simulink model "inv_single_phase"  (R2024b)
settings: Solver=ode1be  StartTime=0.0  StopTime=simlength  FixedStep=ts_sim  MaxStep=ts_sim
undefined symbols (not defined in the file): Adrso, Aresd, Bresd, Cresd, Crso, dead_time, DThs_init, fPWM_INV, freq, frequency_grid, I_FS, ki_i_inv, ki_pll, ki_v_inv, kp_i_inv, kp_pll, kp_v_inv, Ldrso, magnitude, q1kalman, q2kalman, Rkalman, Tambient, ts_inv, ts_zvs, V_FS, w, weigth
libraries: fl_lib x60, nesl_utility x38, ee_lib x9, cstblocks x6
(part 1 of 3)
settings Model: SimulationMode=accelerator  Creator=LTNBDA  LastModifiedBy=dbagn
settings SolverCC: ZeroCrossControl=EnableAll  ZeroCrossAlgorithm=Adaptive  AlgebraicLoopSolver=TrustRegion  SolverResetMethod=Robust  AutoInsertRateTranBlk=on
settings DataIOCC: LimitDataPoints=on  MaxDataPoints=1  SaveFormat=Array  SignalLoggingSaveFormat=ModelDataLogs  SaveOutput=off  SignalLogging=off  DSMLogging=off  SaveTime=off  ReturnWorkspaceOutputs=off
settings OptimizationCC: ExpressionDepthLimit=2147483647  InitFltsAndDblsToZero=on  EfficientMapNaN2IntZero=off  LifeSpan=inf
settings DebuggingCC: SaveWithParameterizedLinksMsg=none  UnderspecifiedInitializationDetection=Classic  MergeDetectMultiDrivingBlocksExec=none  SignalResolutionControl=TryResolveAllWithWarning  SolverPrmCheckMsg=warning  MultiTaskDSMMsg=warning  MultiTaskCondExecSysMsg=none  MultiTaskRateTransMsg=warning  FcnCallInpInsideContextMsg=warning  StateNameClashWarn=warning  SFUnexpectedBacktrackingDiag=warning  SFNoUnconditionalDefaultTransitionDiag=warning  ArithmeticOperatorsInVariantConditions=warning
settings HardwareCC: ProdBitPerLong=64  ProdLargestAtomicFloat=None  ProdIntDivRoundTo=Undefined  ProdEndianess=Unspecified  ProdHWDeviceType=Generic->64-bit Embedded Processor (LP64)  TargetBitPerPointer=64  TargetBitPerSizeT=64  TargetBitPerPtrDiffT=64  TargetLongLongMode=on  TargetIntDivRoundTo=Zero  TargetEndianess=LittleEndian  TargetWordSize=64  TargetHWDeviceType=MATLAB Host  ProdEqTarget=off
settings ModelReferenceCC: EnableRefExpFcnMdlSchedulingChecks=on  PropagateSignalLabelsOutOfModel=off
settings SFSimCC: SimUseLocalCustomCode=off  CustomCodeUndefinedFunction=UseInterfaceOnly
settings RTWCC: RTWUseLocalCustomCode=off  GPUComputeCapability=3.5
settings CodeAppCC: MaxIdLength=128  StateflowObjectComments=on
settings GRTTargetCC: TargetLangStandard=C89/C90 (ANSI)  CombineOutputUpdateFcns=off  GRTInterface=on
settings ConfigComp: CovMetricSettings=dw  CovSaveCumulativeToWorkspaceVar=on  CovSaveSingleToWorkspaceVar=on  CovExternalEMLEnable=off
settings SimscapeCC: SimscapeNormalizeSystem=off

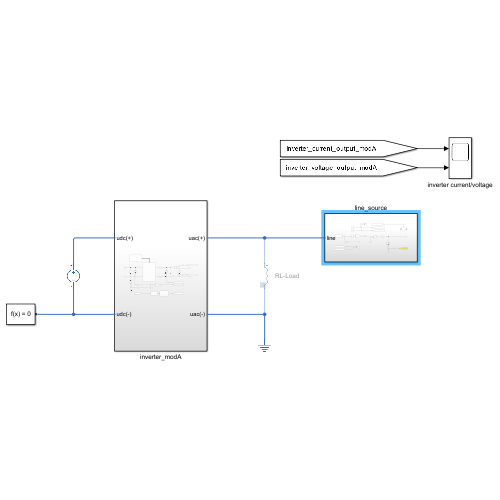
[thumbnail: Simulink's stored preview of the top-level diagram]
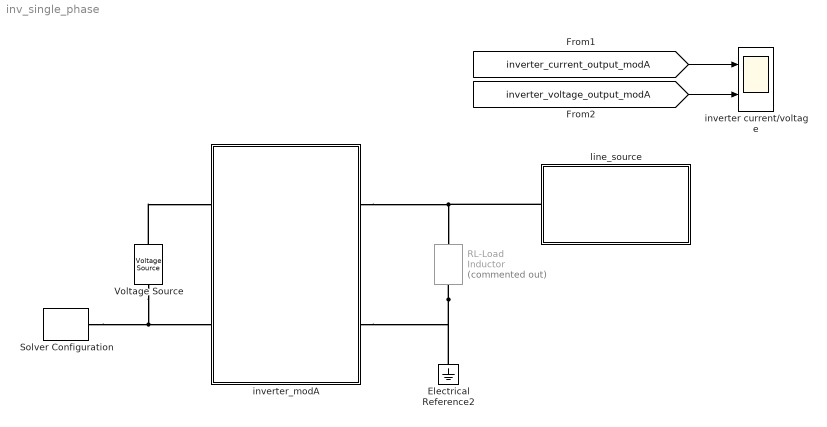
== system inv_single_phase ==
  Electrical Reference2 : fl_lib/Electrical/Electrical Elements/Electrical Reference
  RL-Load : fl_lib/Electrical/Electrical Elements/Inductor  Commented=on  l=Lload H  r=Rload Ohm  g=1e-9 1/Ohm  i_specify=off  i_priority=None  i=0 A  i_nominal_specify=off  i_nominal_value=1  i_nominal_unit=A  v_specify=off  v_priority=None  v=0 V  v_nominal_specify=off  v_nominal_value=1  v_nominal_unit=V  i_L_specify=off  i_L_priority=High  i_L=0 A  i_L_nominal_specify=off  i_L_nominal_value=1  i_L_nominal_unit=A
  Solver Configuration : nesl_utility/Solver Configuration  PhysicalDomain=network_engine_domain  SubClassName=solver  LeftPortType=input  RightPortType=generic  Tones=[]  Harmonics=[]  SimulateNoise=off  Profile=off  UseLocalSampling=off  EnableSwitchedLinearOptims=on  FrequencyDomain=off  UseCCode=off  RelTol=0.001  AbsTol=0.001  MinStep=1e-09  ToWorkspace=off  RevertToSquareIcSolve=off  NumHomotopyIterations=100  PhasorMode=off  PhasorModeNumHarmonics=1  ConsistencySolver=NEWTON_XTOL_AFTER_FTOL  IndexReductionMethod=DerivativeReplacement  DoDC=off  ResidualTolerance=1e-09  ConsistencyTolSource=GLOBAL  ConsistencyAbsTol=0.001  ConsistencyRelTol=0.001  ConsistencyTolFactor=0.001  UseLocalSolver=on  LocalSolverChoice=NE_BACKWARD_EULER_ADVANCER  ResolveIndetEquations=on  FunctionEvalNumThread=1  LocalSolverSampleTime=tc  DoFixedCost=on  MaxNonlinIter=3  MaxModeIter=2  ComputeImpulses=off  ImpulseIterations=2  LinearAlgebra=auto  LinearAlgebraNumThread=0  EquationFormulation=NE_TIME_EF  DelaysMemoryBudget=1024  AutomaticFiltering=on  FilteringTimeConstant=0.001  PartitionStorageMethod=AS_NEEDED  PartitionMemoryBudget=1024  PartitionMethod=ROBUST  MultibodyUseLocalSolver=off  MultibodyLocalSolverChoice=ODE1  MultibodyLocalSolverSampleTime=0.001
  Voltage Source : ee_lib/Sources/Voltage Source  dc_voltage=450 V  ac_voltage=0 V  ac_shift=0 rad  ac_frequency=0 Hz  noise_mode=ee.enum.sources.noise.Disabled  PSD=0 V^2/Hz  sample_time=1e-3 s  repeatability=ee.enum.sources.repeatability.NotRepeatable  user_seed=0  auto_seed=3499211588  i_specify=off  i_priority=None  i=0 A  i_nominal_specify=off  i_nominal_value=1  i_nominal_unit=A  v_specify=off  v_priority=None  v=0 V  v_nominal_specify=off  v_nominal_value=1  v_nominal_unit=V
  inverter current/voltage : Scope  NumInputPorts=2
  inverter_modA : Subsystem
  line_source : Subsystem
  wires:
  [inverter_current_output_modA] -> inverter current/voltage/1
  [inverter_voltage_output_modA] -> inverter current/voltage/2
  connections:
  Voltage Source/RConn1 -- Solver Configuration/RConn1 -- inverter_modA/LConn2
  Voltage Source/LConn1 -- inverter_modA/LConn1
  line_source/LConn1 -- inverter_modA/RConn1 -- RL-Load/LConn1
  RL-Load/RConn1 -- Electrical Reference2/LConn1 -- inverter_modA/RConn2

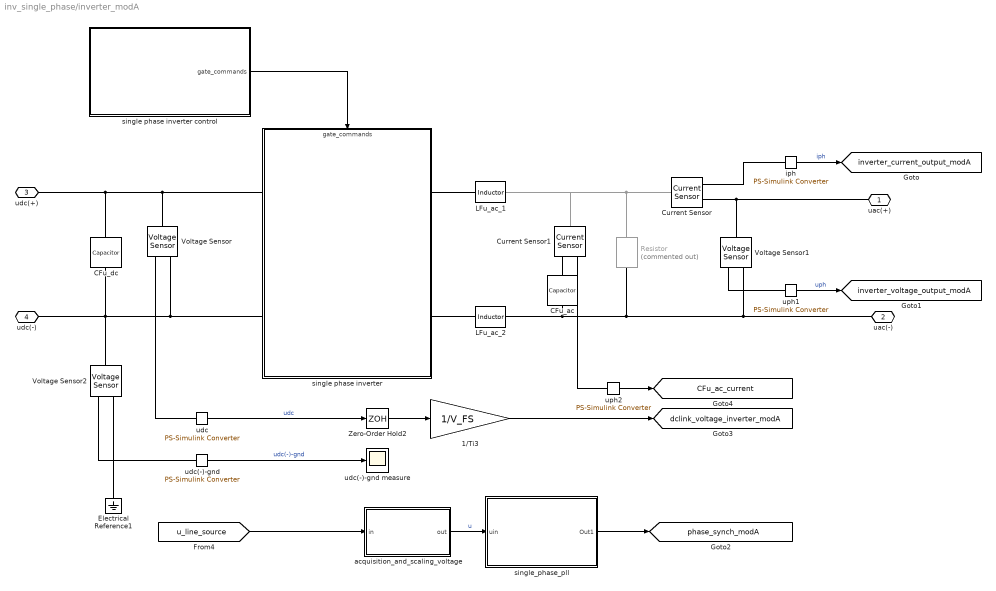
== system inv_single_phase/inverter_modA ==
  1/Ti3 : Gain  Gain=1/V_FS  SaturateOnIntegerOverflow=on  OutDataTypeStr=Inherit: Same as input  ParamDataTypeStr=Inherit: Same as input
  CFu_ac : fl_lib/Electrical/Electrical Elements/Capacitor  c=CFu_ac F  r=RCFu_ac Ohm  g=0 1/Ohm  i_specify=off  i_priority=None  i=0 A  i_nominal_specify=off  i_nominal_value=1  i_nominal_unit=A  v_specify=off  v_priority=None  v=0 V  v_nominal_specify=off  v_nominal_value=1  v_nominal_unit=V  vc_specify=off  vc_priority=High  vc=0 V  vc_nominal_specify=off  vc_nominal_value=1  vc_nominal_unit=V
  CFu_dc : fl_lib/Electrical/Electrical Elements/Capacitor  c=CFu_dc F  r=RCFu_dc_internal Ohm  g=0 1/Ohm  i_specify=off  i_priority=None  i=0 A  i_nominal_specify=off  i_nominal_value=1  i_nominal_unit=A  v_specify=off  v_priority=None  v=0 V  v_nominal_specify=off  v_nominal_value=1  v_nominal_unit=V  vc_specify=off  vc_priority=High  vc=0 V  vc_nominal_specify=off  vc_nominal_value=1  vc_nominal_unit=V
  Current Sensor : fl_lib/Electrical/Electrical Sensors/Current Sensor
  Current Sensor1 : fl_lib/Electrical/Electrical Sensors/Current Sensor
  Electrical Reference1 : fl_lib/Electrical/Electrical Elements/Electrical Reference
  LFu_ac_1 : fl_lib/Electrical/Electrical Elements/Inductor  l=LFu_ac H  r=RLFu_ac Ohm  g=0 1/Ohm  i_specify=on  i_priority=High  i=0 A  i_nominal_specify=off  i_nominal_value=1  i_nominal_unit=A  v_specify=off  v_priority=None  v=0 V  v_nominal_specify=off  v_nominal_value=1  v_nominal_unit=V  i_L_specify=off  i_L_priority=High  i_L=0 A  i_L_nominal_specify=off  i_L_nominal_value=1  i_L_nominal_unit=A
  LFu_ac_2 : fl_lib/Electrical/Electrical Elements/Inductor  l=LFu_ac H  r=RLFu_ac Ohm  g=0 1/Ohm  i_specify=on  i_priority=High  i=0 A  i_nominal_specify=off  i_nominal_value=1  i_nominal_unit=A  v_specify=off  v_priority=None  v=0 V  v_nominal_specify=off  v_nominal_value=1  v_nominal_unit=V  i_L_specify=off  i_L_priority=High  i_L=0 A  i_L_nominal_specify=off  i_L_nominal_value=1  i_L_nominal_unit=A
  Resistor : fl_lib/Electrical/Electrical Elements/Resistor  Commented=on  R=10e3 Ohm  i_specify=off  i_priority=None  i=0 A  i_nominal_specify=off  i_nominal_value=1  i_nominal_unit=A  v_specify=off  v_priority=None  v=0 V  v_nominal_specify=off  v_nominal_value=1  v_nominal_unit=V
  Voltage Sensor : fl_lib/Electrical/Electrical Sensors/Voltage Sensor
  Voltage Sensor1 : fl_lib/Electrical/Electrical Sensors/Voltage Sensor
  Voltage Sensor2 : fl_lib/Electrical/Electrical Sensors/Voltage Sensor
  Zero-Order Hold2 : ZeroOrderHold  SampleTime=ts_zvs
  acquisition_and_scaling_voltage : Subsystem
  iph : nesl_utility/PS-Simulink Converter  PhysicalDomain=network_engine_domain  SubClassName=ps_output  LeftPortType=input  RightPortType=output  PseudoPeriodic=off  Frequencies=[]  VectorFormat=1-D array  Unit=A  AffineConversion=off
  single phase inverter : Subsystem
      settings: PortSchema="{\"entries\":[{\"content\":{\"sides\":[{\"content\":{\"connectorIds\":[\"LConn1\",\"LConn2\"]},\"type\":\"ConnectorPlacement.EquallySpacedRectSide\",\"uuid\":\"4fcf4fea-d38f-431b-8a91-be3ce9782faf\"},{\"content\":{\"connectorIds\":[\"RConn1\",\"RConn2\"],\"side\":\"RIGHT\"},\"type\":\"ConnectorPlacement.EquallySpacedRectSide\",\"uuid\":\"0aa56277-92e9-4e3b-84c7-43398254a4d8\"},{\"content\":{\"connectorIds\":[\"In1\"],\"side\":\"TOP\"},\"type\":\"ConnectorPlacement.EquallySpacedRectSide\",\"uuid\":\"5cd150dc-bcaf-4cd7-b2a8-3db203726730\"}]},\"type\":\"ConnectorPlacement.EquallySpacedConnector\",\"uuid\":\"bf8194c4-c327-4d40-bea4-f1e7617f80b4\"}],\"packageUris\":[\"http://schema.mathworks.com/mf0/Connector/R2020b\"],\"version\":\"1.0\"}"
  single phase inverter control : Subsystem
  single_phase_pll : Subsystem
  udc : nesl_utility/PS-Simulink Converter  PhysicalDomain=network_engine_domain  SubClassName=ps_output  LeftPortType=input  RightPortType=output  PseudoPeriodic=off  Frequencies=[]  VectorFormat=1-D array  Unit=V  AffineConversion=off
  udc(-)-gnd : nesl_utility/PS-Simulink Converter  PhysicalDomain=network_engine_domain  SubClassName=ps_output  LeftPortType=input  RightPortType=output  PseudoPeriodic=off  Frequencies=[]  VectorFormat=1-D array  Unit=V  AffineConversion=off
  udc(-)-gnd measure : Scope
  uph1 : nesl_utility/PS-Simulink Converter  PhysicalDomain=network_engine_domain  SubClassName=ps_output  LeftPortType=input  RightPortType=output  PseudoPeriodic=off  Frequencies=[]  VectorFormat=1-D array  Unit=V  AffineConversion=off
  uph2 : nesl_utility/PS-Simulink Converter  PhysicalDomain=network_engine_domain  SubClassName=ps_output  LeftPortType=input  RightPortType=output  PseudoPeriodic=off  Frequencies=[]  VectorFormat=1-D array  Unit=A  AffineConversion=off
  uac(+) : PMIOPort  Side=Right
  uac(-) : PMIOPort  Port=2  Side=Right
  udc(+) : PMIOPort  Port=3  Side=Left
  udc(-) : PMIOPort  Port=4  Side=Left
  tag scope: CFu_ac_current=global, dclink_voltage_inverter_modA=global, inverter_current_output_modA=global, inverter_voltage_output_modA=global, phase_synch_modA=global
  wires:
  Zero-Order Hold2/1 -> 1/Ti3/1
  1/Ti3/1 -> [dclink_voltage_inverter_modA]
  single phase inverter control/1(gate_commands) -> single phase inverter/1(gate_commands)
  udc/1 -> Zero-Order Hold2/1  "udc"
  iph/1 -> [inverter_current_output_modA]  "iph"
  uph1/1 -> [inverter_voltage_output_modA]  "uph"
  udc(-)-gnd/1 -> udc(-)-gnd measure/1  "udc(-)-gnd"
  uph2/1 -> [CFu_ac_current]
  acquisition_and_scaling_voltage/1(out) -> single_phase_pll/1(uin)  "u"
  [u_line_source] -> acquisition_and_scaling_voltage/1(in)
  single_phase_pll/1(Out1) -> [phase_synch_modA]
  connections:
  single phase inverter/RConn2 -- Voltage Sensor/RConn2 -- CFu_dc/RConn1 -- Voltage Sensor2/LConn1 -- udc(-)/RConn1
  single phase inverter/RConn1 -- CFu_dc/LConn1 -- udc(+)/RConn1 -- Voltage Sensor/LConn1
  LFu_ac_1/LConn1 -- single phase inverter/LConn1
  single phase inverter/LConn2 -- LFu_ac_2/RConn1
  Voltage Sensor/RConn1 -- udc/LConn1
  Voltage Sensor1/RConn1 -- uph1/LConn1
  Resistor/LConn1 -- Current Sensor1/LConn1 -- LFu_ac_1/RConn1 -- Current Sensor/LConn1
  iph/LConn1 -- Current Sensor/RConn1
  uac(+)/RConn1 -- Current Sensor/RConn2 -- Voltage Sensor1/LConn1
  LFu_ac_2/LConn1 -- CFu_ac/RConn1 -- Resistor/RConn1 -- uac(-)/RConn1 -- Voltage Sensor1/RConn2
  Current Sensor1/RConn2 -- CFu_ac/LConn1
  Current Sensor1/RConn1 -- uph2/LConn1
  Voltage Sensor2/RConn1 -- udc(-)-gnd/LConn1
  Electrical Reference1/LConn1 -- Voltage Sensor2/RConn2

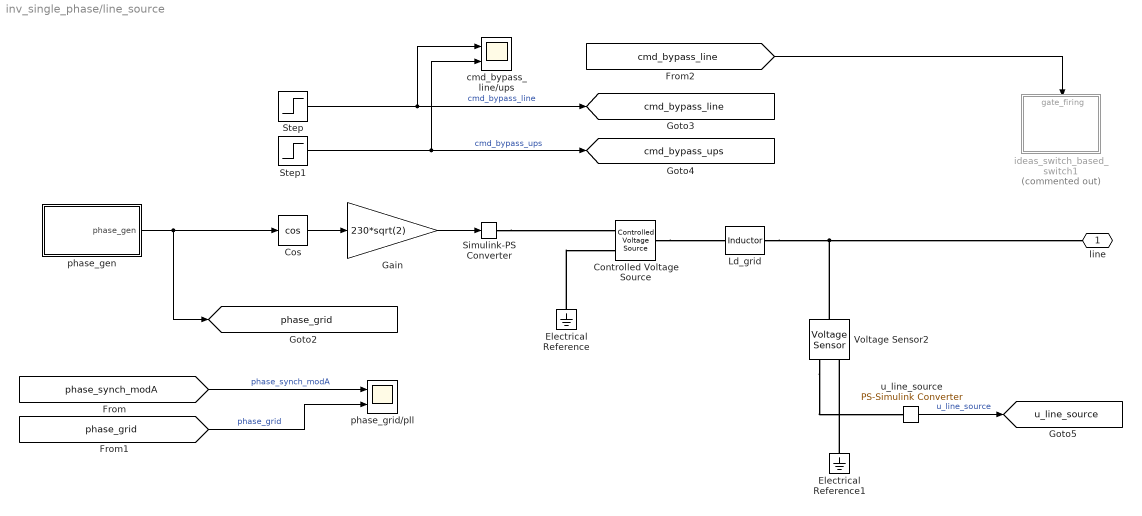
== system inv_single_phase/line_source ==
  Controlled Voltage Source : fl_lib/Electrical/Electrical Sources/Controlled Voltage Source
  Cos : Trigonometry  Operator=cos
  Electrical Reference : fl_lib/Electrical/Electrical Elements/Electrical Reference
  Electrical Reference1 : fl_lib/Electrical/Electrical Elements/Electrical Reference
  Gain : Gain  Gain=230*sqrt(2)
  Ld_grid : fl_lib/Electrical/Electrical Elements/Inductor  l=250e-6 H  r=3e-3 Ohm  g=0 1/Ohm  i_specify=off  i_priority=None  i=0 A  i_nominal_specify=off  i_nominal_value=1  i_nominal_unit=A  v_specify=off  v_priority=None  v=0 V  v_nominal_specify=off  v_nominal_value=1  v_nominal_unit=V  i_L_specify=off  i_L_priority=High  i_L=0 A  i_L_nominal_specify=off  i_L_nominal_value=1  i_L_nominal_unit=A
  Simulink-PS Converter : nesl_utility/Simulink-PS Converter  PhysicalDomain=network_engine_domain  SubClassName=ps_input  LeftPortType=input  RightPortType=output  PseudoPeriodic=off  Frequencies=[]  NoiseDistribution=none  NoiseParameters=[]  Unit=1  AffineConversion=off  FilteringAndDerivatives=provide  SimscapeFilterOrder=1  InputFilterTimeConstant=0.001  UdotUserProvided=0
  Step : Step  Time=0.05  After=15  SampleTime=0
  Step1 : Step  Time=1.2  Before=15  After=0  SampleTime=0
  Voltage Sensor2 : fl_lib/Electrical/Electrical Sensors/Voltage Sensor
  cmd_bypass_line/ups : Scope  NumInputPorts=2
  ideas_switch_based_switch1 : Subsystem  Commented=on
      settings: PortSchema="{\"entries\":[{\"content\":{\"sides\":[{\"content\":{\"connectorIds\":[\"LConn1\"]},\"type\":\"ConnectorPlacement.EquallySpacedRectSide\",\"uuid\":\"0c1d3d49-2b2f-458b-aa4f-29a8fc7e06a8\"},{\"content\":{\"connectorIds\":[\"RConn1\"],\"side\":\"RIGHT\"},\"type\":\"ConnectorPlacement.EquallySpacedRectSide\",\"uuid\":\"ca3eb42d-18fc-4989-b764-44975cb49bad\"},{\"content\":{\"connectorIds\":[\"In1\"],\"side\":\"TOP\"},\"type\":\"ConnectorPlacement.EquallySpacedRectSide\",\"uuid\":\"521c1188-cf36-48df-a46f-4a5e2a9fee19\"}]},\"type\":\"ConnectorPlacement.EquallySpacedConnector\",\"uuid\":\"019ba21c-6ae7-40bf-b23d-41e1cbba37d5\"}],\"packageUris\":[\"http://schema.mathworks.com/mf0/Connector/R2020b\"],\"version\":\"1.0\"}"
  phase_gen : Subsystem
  phase_grid/pll : Scope  NumInputPorts=2
  u_line_source : nesl_utility/PS-Simulink Converter  PhysicalDomain=network_engine_domain  SubClassName=ps_output  LeftPortType=input  RightPortType=output  PseudoPeriodic=off  Frequencies=[]  VectorFormat=1-D array  Unit=V  AffineConversion=off
  line : PMIOPort  Side=Left
  tag scope: cmd_bypass_line=global, cmd_bypass_ups=global, phase_grid=global, u_line_source=global
  wires:
  phase_gen/1(phase_gen) -> Cos/1, [phase_grid]
  Step1/1 -> cmd_bypass_line/ups/2, [cmd_bypass_ups]  "cmd_bypass_ups"
  Step/1 -> cmd_bypass_line/ups/1, [cmd_bypass_line]  "cmd_bypass_line"
  Cos/1 -> Gain/1
  Gain/1 -> Simulink-PS Converter/1
  [phase_synch_modA] -> phase_grid/pll/1  "phase_synch_modA"
  [phase_grid] -> phase_grid/pll/2  "phase_grid"
  [cmd_bypass_line] -> ideas_switch_based_switch1/1(gate_firing)
  u_line_source/1 -> [u_line_source]  "u_line_source"
  connections:
  Simulink-PS Converter/RConn1 -- Controlled Voltage Source/RConn1
  Electrical Reference/LConn1 -- Controlled Voltage Source/RConn2
  Controlled Voltage Source/LConn1 -- Ld_grid/LConn1
  Ld_grid/RConn1 -- line/RConn1 -- Voltage Sensor2/LConn1
  Electrical Reference1/LConn1 -- Voltage Sensor2/RConn2
  Voltage Sensor2/RConn1 -- u_line_source/LConn1

== system inv_single_phase/inverter_modA/acquisition_and_scaling_voltage ==
  in : Inport
  1/Ti1 : Gain  Gain=1/V_FS  SaturateOnIntegerOverflow=on  OutDataTypeStr=Inherit: Same as input  ParamDataTypeStr=Inherit: Same as input
  Unit Delay4 : UnitDelay  SampleTime=ts_inv  HasFrameUpgradeWarning=on
  Zero-Order Hold2 : ZeroOrderHold  SampleTime=ts_inv
  out : Outport
  wires:
  1/Ti1/1 -> Unit Delay4/1
  Zero-Order Hold2/1 -> 1/Ti1/1
  Unit Delay4/1 -> out/1
  in/1 -> Zero-Order Hold2/1

== system inv_single_phase/inverter_modA/single phase inverter ==
  gate_commands : Inport
  Current Sensor : fl_lib/Electrical/Electrical Sensors/Current Sensor
  HBridgeIdeal : Subsystem
  HBridgeMosfet : Subsystem  Commented=on
  HBridgeThermal : Subsystem  Commented=on
  Voltage Sensor1 : fl_lib/Electrical/Electrical Sensors/Voltage Sensor
  iph : nesl_utility/PS-Simulink Converter  PhysicalDomain=network_engine_domain  SubClassName=ps_output  LeftPortType=input  RightPortType=output  PseudoPeriodic=off  Frequencies=[]  VectorFormat=1-D array  Unit=A  AffineConversion=off
  uph1 : nesl_utility/PS-Simulink Converter  PhysicalDomain=network_engine_domain  SubClassName=ps_output  LeftPortType=input  RightPortType=output  PseudoPeriodic=off  Frequencies=[]  VectorFormat=1-D array  Unit=V  AffineConversion=off
  uac_out(+) : PMIOPort  Side=Left
  uac_out(-) : PMIOPort  Port=2  Side=Left
  udc(+) : PMIOPort  Port=3  Side=Right
  udc(-) : PMIOPort  Port=4  Side=Right
  tag scope: is_inv_modA=global, us_inv_modA=global
  wires:
  iph/1 -> [is_inv_modA]  "iph"
  uph1/1 -> [us_inv_modA]  "uph"
  gate_commands/1 -> HBridgeIdeal/1(gate_commands)
  connections:
  Current Sensor/RConn1 -- iph/LConn1
  Current Sensor/RConn2 -- Voltage Sensor1/LConn1 -- uac_out(+)/RConn1
  Voltage Sensor1/RConn1 -- uph1/LConn1
  Voltage Sensor1/RConn2 -- HBridgeIdeal/RConn2 -- uac_out(-)/RConn1
  HBridgeIdeal/LConn1 -- udc(+)/RConn1
  HBridgeIdeal/RConn1 -- Current Sensor/LConn1
  HBridgeIdeal/LConn2 -- udc(-)/RConn1

== system inv_single_phase/inverter_modA/single phase inverter control ==
  Bus Creator : BusCreator  Inputs=4
  Bus Creator1 : BusCreator  Inputs=2
  Bus Creator2 : BusCreator  Inputs=2
  acquisition_and_scaling_current : Subsystem
  acquisition_and_scaling_voltage : Subsystem
  dqbased_single_phase_inverter_ctrl : Subsystem  Commented=on
  is/is_ref : Scope  NumInputPorts=2
  pwm : Subsystem
  references_generator : Subsystem
  rpi_based_single_phase_inverter_ctrl : Subsystem
  gate_commands : Outport
  wires:
  pwm/3(m2_top) -> Bus Creator/3
  Bus Creator/1 -> gate_commands/1
  pwm/1(m1_top) -> Bus Creator/1
  pwm/2(m1_bottom) -> Bus Creator/2
  pwm/4(m2_bottom) -> Bus Creator/4
  [is_inv_modA] -> acquisition_and_scaling_current/1(in)
  [inverter_voltage_output_modA] -> acquisition_and_scaling_voltage/1(in)
  acquisition_and_scaling_current/1(out) -> Bus Creator1/1, rpi_based_single_phase_inverter_ctrl/1(i_out_inverter_pu)  "is_pu"
  acquisition_and_scaling_voltage/1(out) -> rpi_based_single_phase_inverter_ctrl/2(u_out_inverter_pu)  "u_out_inverter_pu"
  rpi_based_single_phase_inverter_ctrl/1(u_ctrl_out) -> pwm/1(vout)
  references_generator/1(i_out_inverter_reference_pu) -> Bus Creator1/2, rpi_based_single_phase_inverter_ctrl/3(i_out_inverter_reference_pu)  "is_ref_pu"
  references_generator/2(u_out_inverter_reference_pu) -> rpi_based_single_phase_inverter_ctrl/4(u_out_inverter_reference_pu)  "u_out_inverter_reference_pu"
  Bus Creator1/1 -> is/is_ref/2  "is_tracking"
  [is_inv_modA] -> Bus Creator2/2  "is"
  Bus Creator2/1 -> is/is_ref/1  "load"
  [inverter_voltage_output_modA] -> Bus Creator2/1  "u_out"

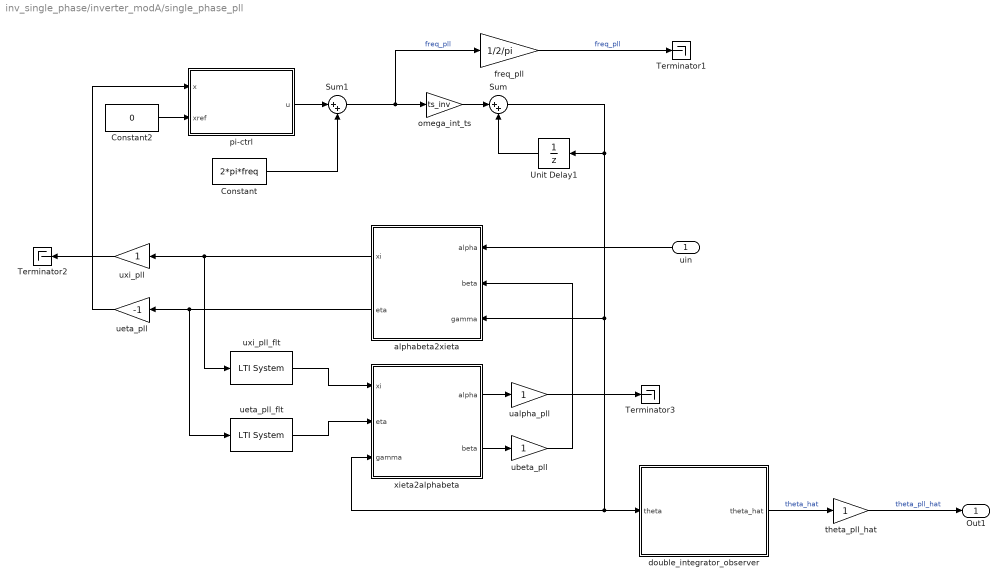
== system inv_single_phase/inverter_modA/single_phase_pll ==
  uin : Inport
  Constant : Constant  Value=2*pi*freq
  Constant2 : Constant  Value=0
  Sum : Sum  Inputs=|++
  Sum1 : Sum  Inputs=|++
  Terminator1 : Terminator
  Terminator2 : Terminator
  Terminator3 : Terminator
  Unit Delay1 : UnitDelay  SampleTime=ts_inv  HasFrameUpgradeWarning=on
  alphabeta2xieta : MATLAB Function  TreatAsAtomicUnit=on  SystemSampleTime=ts_inv
  double_integrator_observer : Subsystem
  freq_pll : Gain  Gain=1/2/pi
  omega_int_ts : Gain  Gain=ts_inv
  pi-ctrl : Subsystem  mask{kp=kp_pll, ki=ki_pll, ts=ts_inv, sat_pos=inf, sat_neg=-inf}
  theta_pll_hat : Gain
  ualpha_pll : Gain
  ubeta_pll : Gain
  ueta_pll : Gain  Gain=-1
  ueta_pll_flt : cstblocks/LTI System  sys=Hd  IC=[]  PadeOrder=0
  uxi_pll : Gain
  uxi_pll_flt : cstblocks/LTI System  sys=Hd  IC=[]  PadeOrder=0
  xieta2alphabeta : MATLAB Function  TreatAsAtomicUnit=on  SystemSampleTime=ts_inv
  Out1 : Outport
  wires:
  Sum/1 -> double_integrator_observer/1(theta), xieta2alphabeta/3(gamma), alphabeta2xieta/3(gamma), Unit Delay1/1
  Unit Delay1/1 -> Sum/2
  alphabeta2xieta/1(xi) -> uxi_pll_flt/1, uxi_pll/1
  xieta2alphabeta/2(beta) -> ubeta_pll/1
  alphabeta2xieta/2(eta) -> ueta_pll_flt/1, ueta_pll/1
  omega_int_ts/1 -> Sum/1
  double_integrator_observer/1(theta_hat) -> theta_pll_hat/1  "theta_hat"
  uin/1 -> alphabeta2xieta/1(alpha)
  freq_pll/1 -> Terminator1/1  "freq_pll"
  ueta_pll_flt/1 -> xieta2alphabeta/2(eta)
  uxi_pll_flt/1 -> xieta2alphabeta/1(xi)
  ueta_pll/1 -> pi-ctrl/1(x)
  Sum1/1 -> freq_pll/1, omega_int_ts/1  "freq_pll"
  Constant2/1 -> pi-ctrl/2(xref)
  uxi_pll/1 -> Terminator2/1
  ubeta_pll/1 -> alphabeta2xieta/2(beta)
  xieta2alphabeta/1(alpha) -> ualpha_pll/1
  ualpha_pll/1 -> Terminator3/1
  pi-ctrl/1(u) -> Sum1/1
  Constant/1 -> Sum1/2
  theta_pll_hat/1 -> Out1/1  "theta_pll_hat"

== system inv_single_phase/line_source/ideas_switch_based_switch1 ==
  gate_firing : Inport
  Simulink-PS Converter : nesl_utility/Simulink-PS Converter  PhysicalDomain=network_engine_domain  SubClassName=ps_input  LeftPortType=input  RightPortType=output  PseudoPeriodic=off  Frequencies=[]  NoiseDistribution=none  NoiseParameters=[]  Unit=1  AffineConversion=off  FilteringAndDerivatives=provide  SimscapeFilterOrder=1  InputFilterTimeConstant=0.001  UdotUserProvided=0
  Switch : fl_lib/Electrical/Electrical Elements/Switch  R_closed=Ron Ohm  G_open=1e-8 1/Ohm  Threshold=7.5  i_specify=off  i_priority=None  i=0 A  i_nominal_specify=off  i_nominal_value=1  i_nominal_unit=A  v_specify=off  v_priority=None  v=0 V  v_nominal_specify=off  v_nominal_value=1  v_nominal_unit=V
  u1 : PMIOPort  Side=Left
  u2 : PMIOPort  Port=2  Side=Right
  wires:
  gate_firing/1 -> Simulink-PS Converter/1
  connections:
  Simulink-PS Converter/RConn1 -- Switch/RConn1
  Switch/LConn1 -- u2/RConn1
  u1/RConn1 -- Switch/RConn2

== system inv_single_phase/line_source/phase_gen ==
  Constant4 : Constant  Value=2*pi*frequency_grid
  Sum4 : Sum  SaturateOnIntegerOverflow=on
  Unit Delay1 : UnitDelay  SampleTime=ts_inv  HasFrameUpgradeWarning=on
  bounder1 : MATLAB Function  TreatAsAtomicUnit=on  SystemSampleTime=ts_inv
  kp2 : Gain  Gain=ts_inv  SaturateOnIntegerOverflow=on  OutDataTypeStr=Inherit: Same as input  ParamDataTypeStr=Inherit: Same as input
  phase_gen : Outport  VectorParamsAs1DForOutWhenUnconnected=off
  wires:
  bounder1/1(y) -> Unit Delay1/1  "grid_emu_phase"
  kp2/1 -> Sum4/1
  Constant4/1 -> kp2/1
  Unit Delay1/1 -> Sum4/2, phase_gen/1
  Sum4/1 -> bounder1/1(u)

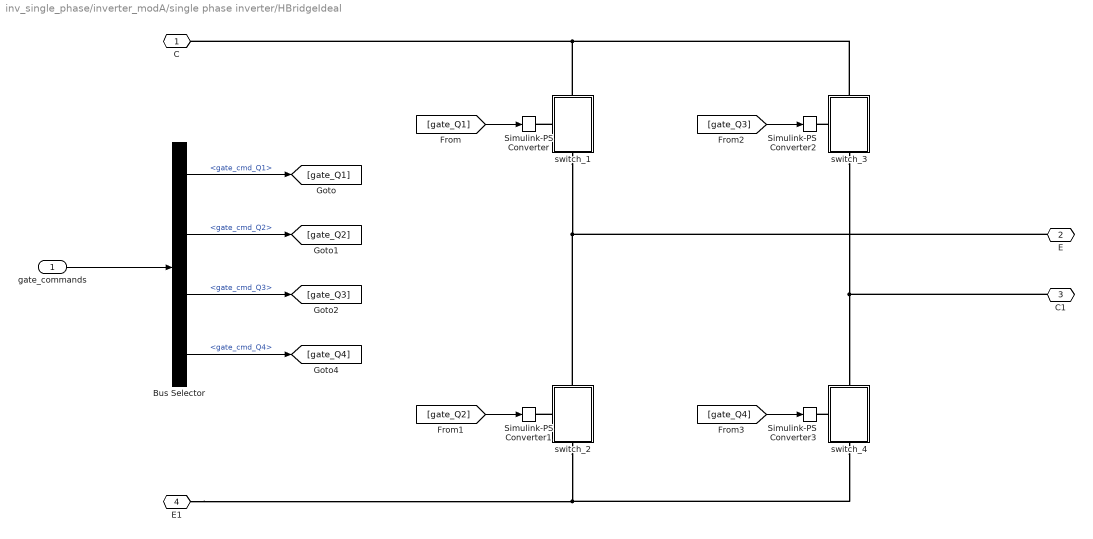
== system inv_single_phase/inverter_modA/single phase inverter/HBridgeIdeal ==
  gate_commands : Inport
  Bus Selector : BusSelector  OutputSignals=gate_cmd_Q1,gate_cmd_Q2,gate_cmd_Q3,gate_cmd_Q4
  Simulink-PS Converter{,1..3} (4 alike) : nesl_utility/Simulink-PS Converter  PhysicalDomain=network_engine_domain  SubClassName=ps_input  LeftPortType=input  RightPortType=output  PseudoPeriodic=off  Frequencies=[]  NoiseDistribution=none  NoiseParameters=[]  Unit=1  AffineConversion=on  FilteringAndDerivatives=provide  SimscapeFilterOrder=1  InputFilterTimeConstant=0.001  UdotUserProvided=0
  switch_1 : Subsystem
      settings: PortSchema="{\"entries\":[{\"content\":{\"sides\":[{\"content\":{\"connectorIds\":[\"LConn1\"]},\"type\":\"ConnectorPlacement.EquallySpacedRectSide\",\"uuid\":\"9277da8d-d460-43e6-8478-dd662f15d226\"},{\"content\":{\"connectorIds\":[],\"side\":\"RIGHT\"},\"type\":\"ConnectorPlacement.EquallySpacedRectSide\",\"uuid\":\"a7ece396-f1d9-4f4f-a05b-db1fc65d6e1d\"},{\"content\":{\"connectorIds\":[\"LConn2\"],\"side\":\"TOP\"},\"type\":\"ConnectorPlacement.EquallySpacedRectSide\",\"uuid\":\"fdd70777-e9cf-4317-afb6-cae87f75d5b0\"},{\"content\":{\"connectorIds\":[\"RConn1\"],\"side\":\"BOTTOM\"},\"type\":\"ConnectorPlacement.EquallySpacedRectSide\",\"uuid\":\"2353ed68-b1a1-4775-9ca9-31e268d5443b\"}]},\"type\":\"ConnectorPlacement.EquallySpacedConnector\",\"uuid\":\"d5479f4c-4e65-4791-adcb-73df11f88590\"}],\"packageUris\":[\"http://schema.mathworks.com/mf0/Connector/R2020b\"],\"version\":\"1.0\"}"
  switch_2 : Subsystem
      settings: PortSchema="{\"entries\":[{\"content\":{\"sides\":[{\"content\":{\"connectorIds\":[\"LConn1\"]},\"type\":\"ConnectorPlacement.EquallySpacedRectSide\",\"uuid\":\"9277da8d-d460-43e6-8478-dd662f15d226\"},{\"content\":{\"connectorIds\":[],\"side\":\"RIGHT\"},\"type\":\"ConnectorPlacement.EquallySpacedRectSide\",\"uuid\":\"a7ece396-f1d9-4f4f-a05b-db1fc65d6e1d\"},{\"content\":{\"connectorIds\":[\"LConn2\"],\"side\":\"TOP\"},\"type\":\"ConnectorPlacement.EquallySpacedRectSide\",\"uuid\":\"fdd70777-e9cf-4317-afb6-cae87f75d5b0\"},{\"content\":{\"connectorIds\":[\"RConn1\"],\"side\":\"BOTTOM\"},\"type\":\"ConnectorPlacement.EquallySpacedRectSide\",\"uuid\":\"2353ed68-b1a1-4775-9ca9-31e268d5443b\"}]},\"type\":\"ConnectorPlacement.EquallySpacedConnector\",\"uuid\":\"d5479f4c-4e65-4791-adcb-73df11f88590\"}],\"packageUris\":[\"http://schema.mathworks.com/mf0/Connector/R2020b\"],\"version\":\"1.0\"}"
  switch_3 : Subsystem
      settings: PortSchema="{\"entries\":[{\"content\":{\"sides\":[{\"content\":{\"connectorIds\":[\"LConn1\"]},\"type\":\"ConnectorPlacement.EquallySpacedRectSide\",\"uuid\":\"9277da8d-d460-43e6-8478-dd662f15d226\"},{\"content\":{\"connectorIds\":[],\"side\":\"RIGHT\"},\"type\":\"ConnectorPlacement.EquallySpacedRectSide\",\"uuid\":\"a7ece396-f1d9-4f4f-a05b-db1fc65d6e1d\"},{\"content\":{\"connectorIds\":[\"LConn2\"],\"side\":\"TOP\"},\"type\":\"ConnectorPlacement.EquallySpacedRectSide\",\"uuid\":\"fdd70777-e9cf-4317-afb6-cae87f75d5b0\"},{\"content\":{\"connectorIds\":[\"RConn1\"],\"side\":\"BOTTOM\"},\"type\":\"ConnectorPlacement.EquallySpacedRectSide\",\"uuid\":\"2353ed68-b1a1-4775-9ca9-31e268d5443b\"}]},\"type\":\"ConnectorPlacement.EquallySpacedConnector\",\"uuid\":\"d5479f4c-4e65-4791-adcb-73df11f88590\"}],\"packageUris\":[\"http://schema.mathworks.com/mf0/Connector/R2020b\"],\"version\":\"1.0\"}"
  switch_4 : Subsystem
      settings: PortSchema="{\"entries\":[{\"content\":{\"sides\":[{\"content\":{\"connectorIds\":[\"LConn1\"]},\"type\":\"ConnectorPlacement.EquallySpacedRectSide\",\"uuid\":\"9277da8d-d460-43e6-8478-dd662f15d226\"},{\"content\":{\"connectorIds\":[],\"side\":\"RIGHT\"},\"type\":\"ConnectorPlacement.EquallySpacedRectSide\",\"uuid\":\"a7ece396-f1d9-4f4f-a05b-db1fc65d6e1d\"},{\"content\":{\"connectorIds\":[\"LConn2\"],\"side\":\"TOP\"},\"type\":\"ConnectorPlacement.EquallySpacedRectSide\",\"uuid\":\"fdd70777-e9cf-4317-afb6-cae87f75d5b0\"},{\"content\":{\"connectorIds\":[\"RConn1\"],\"side\":\"BOTTOM\"},\"type\":\"ConnectorPlacement.EquallySpacedRectSide\",\"uuid\":\"2353ed68-b1a1-4775-9ca9-31e268d5443b\"}]},\"type\":\"ConnectorPlacement.EquallySpacedConnector\",\"uuid\":\"d5479f4c-4e65-4791-adcb-73df11f88590\"}],\"packageUris\":[\"http://schema.mathworks.com/mf0/Connector/R2020b\"],\"version\":\"1.0\"}"
  C : PMIOPort  Side=Left
  E : PMIOPort  Port=2  Side=Right
  C1 : PMIOPort  Port=3  Side=Right
  E1 : PMIOPort  Port=4  Side=Left
  wires:
  [gate_Q3] -> Simulink-PS Converter2/1
  Bus Selector/2 -> [gate_Q2]  "<gate_cmd_Q2>"
  Bus Selector/1 -> [gate_Q1]  "<gate_cmd_Q1>"
  Bus Selector/3 -> [gate_Q3]  "<gate_cmd_Q3>"
  [gate_Q4] -> Simulink-PS Converter3/1
  [gate_Q2] -> Simulink-PS Converter1/1
  [gate_Q1] -> Simulink-PS Converter/1
  Bus Selector/4 -> [gate_Q4]  "<gate_cmd_Q4>"
  gate_commands/1 -> Bus Selector/1
  connections:
  switch_1/LConn1 -- Simulink-PS Converter/RConn1
  switch_3/LConn2 -- C/RConn1 -- switch_1/LConn2
  switch_4/RConn1 -- E1/RConn1 -- switch_2/RConn1
  switch_2/LConn2 -- switch_1/RConn1 -- E/RConn1
  switch_3/LConn1 -- Simulink-PS Converter2/RConn1
  switch_3/RConn1 -- switch_4/LConn2 -- C1/RConn1
  switch_2/LConn1 -- Simulink-PS Converter1/RConn1
  switch_4/LConn1 -- Simulink-PS Converter3/RConn1

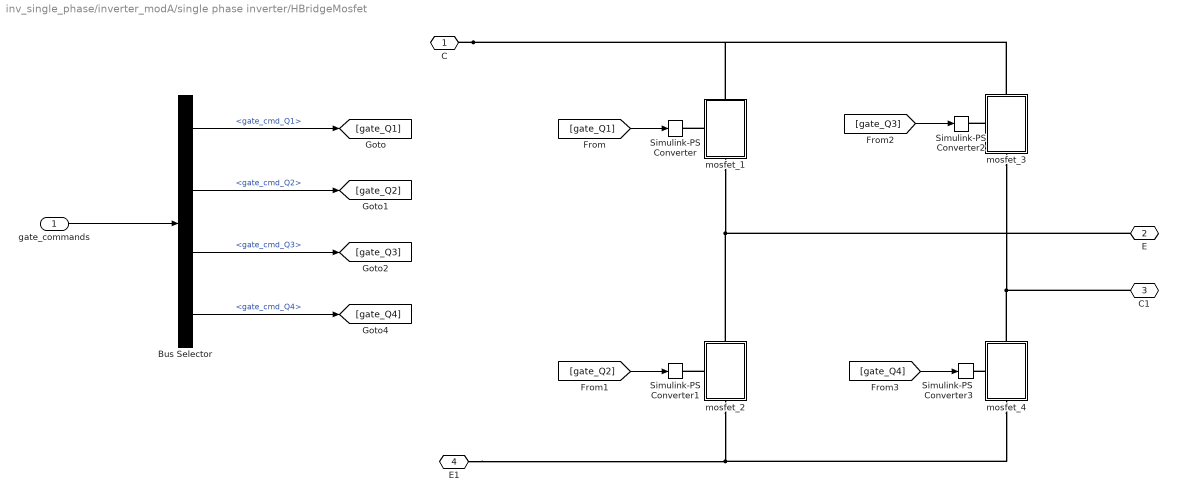
== system inv_single_phase/inverter_modA/single phase inverter/HBridgeMosfet ==
  gate_commands : Inport
  Bus Selector : BusSelector  OutputSignals=gate_cmd_Q1,gate_cmd_Q2,gate_cmd_Q3,gate_cmd_Q4
  Simulink-PS Converter{,1..3} (4 alike) : nesl_utility/Simulink-PS Converter  PhysicalDomain=network_engine_domain  SubClassName=ps_input  LeftPortType=input  RightPortType=output  PseudoPeriodic=off  Frequencies=[]  NoiseDistribution=none  NoiseParameters=[]  Unit=V  AffineConversion=off  FilteringAndDerivatives=provide  SimscapeFilterOrder=1  InputFilterTimeConstant=0.001  UdotUserProvided=0
  mosfet_1 : Subsystem
      settings: PortSchema="{\"entries\":[{\"content\":{\"sides\":[{\"content\":{\"connectorIds\":[\"LConn1\"]},\"type\":\"ConnectorPlacement.EquallySpacedRectSide\",\"uuid\":\"9277da8d-d460-43e6-8478-dd662f15d226\"},{\"content\":{\"connectorIds\":[],\"side\":\"RIGHT\"},\"type\":\"ConnectorPlacement.EquallySpacedRectSide\",\"uuid\":\"a7ece396-f1d9-4f4f-a05b-db1fc65d6e1d\"},{\"content\":{\"connectorIds\":[\"LConn2\"],\"side\":\"TOP\"},\"type\":\"ConnectorPlacement.EquallySpacedRectSide\",\"uuid\":\"fdd70777-e9cf-4317-afb6-cae87f75d5b0\"},{\"content\":{\"connectorIds\":[\"RConn1\"],\"side\":\"BOTTOM\"},\"type\":\"ConnectorPlacement.EquallySpacedRectSide\",\"uuid\":\"2353ed68-b1a1-4775-9ca9-31e268d5443b\"}]},\"type\":\"ConnectorPlacement.EquallySpacedConnector\",\"uuid\":\"d5479f4c-4e65-4791-adcb-73df11f88590\"}],\"packageUris\":[\"http://schema.mathworks.com/mf0/Connector/R2020b\"],\"version\":\"1.0\"}"
  mosfet_2 : Subsystem
      settings: PortSchema="{\"entries\":[{\"content\":{\"sides\":[{\"content\":{\"connectorIds\":[\"LConn1\"]},\"type\":\"ConnectorPlacement.EquallySpacedRectSide\",\"uuid\":\"9277da8d-d460-43e6-8478-dd662f15d226\"},{\"content\":{\"connectorIds\":[],\"side\":\"RIGHT\"},\"type\":\"ConnectorPlacement.EquallySpacedRectSide\",\"uuid\":\"a7ece396-f1d9-4f4f-a05b-db1fc65d6e1d\"},{\"content\":{\"connectorIds\":[\"LConn2\"],\"side\":\"TOP\"},\"type\":\"ConnectorPlacement.EquallySpacedRectSide\",\"uuid\":\"fdd70777-e9cf-4317-afb6-cae87f75d5b0\"},{\"content\":{\"connectorIds\":[\"RConn1\"],\"side\":\"BOTTOM\"},\"type\":\"ConnectorPlacement.EquallySpacedRectSide\",\"uuid\":\"2353ed68-b1a1-4775-9ca9-31e268d5443b\"}]},\"type\":\"ConnectorPlacement.EquallySpacedConnector\",\"uuid\":\"d5479f4c-4e65-4791-adcb-73df11f88590\"}],\"packageUris\":[\"http://schema.mathworks.com/mf0/Connector/R2020b\"],\"version\":\"1.0\"}"
  mosfet_3 : Subsystem
      settings: PortSchema="{\"entries\":[{\"content\":{\"sides\":[{\"content\":{\"connectorIds\":[\"LConn1\"]},\"type\":\"ConnectorPlacement.EquallySpacedRectSide\",\"uuid\":\"9277da8d-d460-43e6-8478-dd662f15d226\"},{\"content\":{\"connectorIds\":[],\"side\":\"RIGHT\"},\"type\":\"ConnectorPlacement.EquallySpacedRectSide\",\"uuid\":\"a7ece396-f1d9-4f4f-a05b-db1fc65d6e1d\"},{\"content\":{\"connectorIds\":[\"LConn2\"],\"side\":\"TOP\"},\"type\":\"ConnectorPlacement.EquallySpacedRectSide\",\"uuid\":\"fdd70777-e9cf-4317-afb6-cae87f75d5b0\"},{\"content\":{\"connectorIds\":[\"RConn1\"],\"side\":\"BOTTOM\"},\"type\":\"ConnectorPlacement.EquallySpacedRectSide\",\"uuid\":\"2353ed68-b1a1-4775-9ca9-31e268d5443b\"}]},\"type\":\"ConnectorPlacement.EquallySpacedConnector\",\"uuid\":\"d5479f4c-4e65-4791-adcb-73df11f88590\"}],\"packageUris\":[\"http://schema.mathworks.com/mf0/Connector/R2020b\"],\"version\":\"1.0\"}"
  mosfet_4 : Subsystem
      settings: PortSchema="{\"entries\":[{\"content\":{\"sides\":[{\"content\":{\"connectorIds\":[\"LConn1\"]},\"type\":\"ConnectorPlacement.EquallySpacedRectSide\",\"uuid\":\"9277da8d-d460-43e6-8478-dd662f15d226\"},{\"content\":{\"connectorIds\":[],\"side\":\"RIGHT\"},\"type\":\"ConnectorPlacement.EquallySpacedRectSide\",\"uuid\":\"a7ece396-f1d9-4f4f-a05b-db1fc65d6e1d\"},{\"content\":{\"connectorIds\":[\"LConn2\"],\"side\":\"TOP\"},\"type\":\"ConnectorPlacement.EquallySpacedRectSide\",\"uuid\":\"fdd70777-e9cf-4317-afb6-cae87f75d5b0\"},{\"content\":{\"connectorIds\":[\"RConn1\"],\"side\":\"BOTTOM\"},\"type\":\"ConnectorPlacement.EquallySpacedRectSide\",\"uuid\":\"2353ed68-b1a1-4775-9ca9-31e268d5443b\"}]},\"type\":\"ConnectorPlacement.EquallySpacedConnector\",\"uuid\":\"d5479f4c-4e65-4791-adcb-73df11f88590\"}],\"packageUris\":[\"http://schema.mathworks.com/mf0/Connector/R2020b\"],\"version\":\"1.0\"}"
  C : PMIOPort  Side=Left
  E : PMIOPort  Port=2  Side=Right
  C1 : PMIOPort  Port=3  Side=Right
  E1 : PMIOPort  Port=4  Side=Left
  wires:
  [gate_Q3] -> Simulink-PS Converter2/1
  Bus Selector/2 -> [gate_Q2]  "<gate_cmd_Q2>"
  Bus Selector/1 -> [gate_Q1]  "<gate_cmd_Q1>"
  Bus Selector/3 -> [gate_Q3]  "<gate_cmd_Q3>"
  [gate_Q4] -> Simulink-PS Converter3/1
  [gate_Q2] -> Simulink-PS Converter1/1
  [gate_Q1] -> Simulink-PS Converter/1
  Bus Selector/4 -> [gate_Q4]  "<gate_cmd_Q4>"
  gate_commands/1 -> Bus Selector/1
  connections:
  mosfet_1/LConn1 -- Simulink-PS Converter/RConn1
  C/RConn1 -- mosfet_3/LConn2 -- mosfet_1/LConn2
  E1/RConn1 -- mosfet_4/RConn1 -- mosfet_2/RConn1
  E/RConn1 -- mosfet_2/LConn2 -- mosfet_1/RConn1
  mosfet_3/LConn1 -- Simulink-PS Converter2/RConn1
  C1/RConn1 -- mosfet_4/LConn2 -- mosfet_3/RConn1
  mosfet_2/LConn1 -- Simulink-PS Converter1/RConn1
  mosfet_4/LConn1 -- Simulink-PS Converter3/RConn1

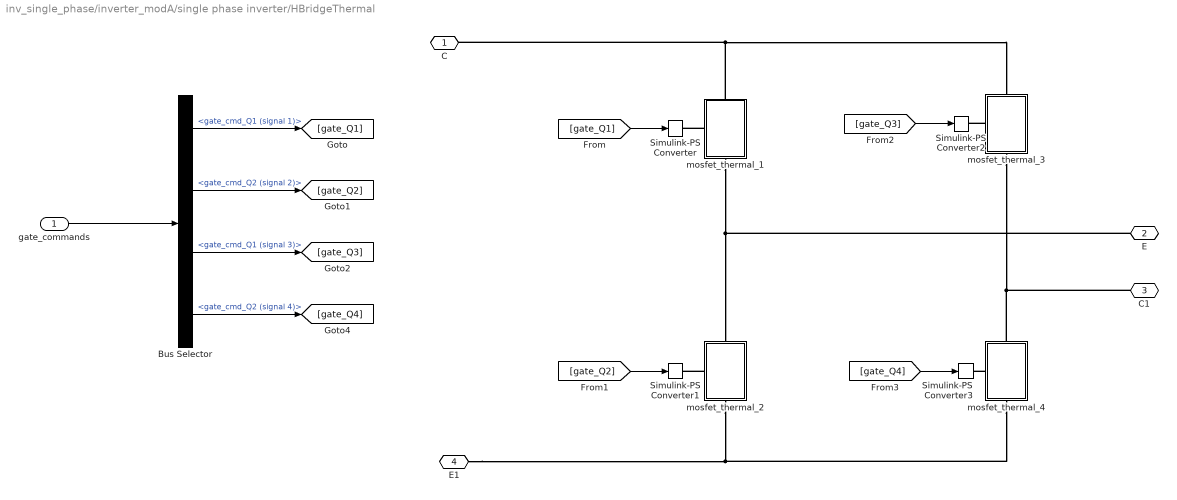
== system inv_single_phase/inverter_modA/single phase inverter/HBridgeThermal ==
  gate_commands : Inport
  Bus Selector : BusSelector  OutputSignals=gate_cmd_Q1 (signal 1),gate_cmd_Q2 (signal 2),gate_cmd_Q1 (signal 3),gate_cmd_Q2 (signal 4)
  Simulink-PS Converter{,1..3} (4 alike) : nesl_utility/Simulink-PS Converter  PhysicalDomain=network_engine_domain  SubClassName=ps_input  LeftPortType=input  RightPortType=output  PseudoPeriodic=off  Frequencies=[]  NoiseDistribution=none  NoiseParameters=[]  Unit=V  AffineConversion=off  FilteringAndDerivatives=provide  SimscapeFilterOrder=1  InputFilterTimeConstant=0.001  UdotUserProvided=0
  mosfet_thermal_1 : Subsystem
      settings: PortSchema="{\"entries\":[{\"content\":{\"sides\":[{\"content\":{\"connectorIds\":[\"LConn1\"]},\"type\":\"ConnectorPlacement.EquallySpacedRectSide\",\"uuid\":\"9277da8d-d460-43e6-8478-dd662f15d226\"},{\"content\":{\"connectorIds\":[],\"side\":\"RIGHT\"},\"type\":\"ConnectorPlacement.EquallySpacedRectSide\",\"uuid\":\"a7ece396-f1d9-4f4f-a05b-db1fc65d6e1d\"},{\"content\":{\"connectorIds\":[\"LConn2\"],\"side\":\"TOP\"},\"type\":\"ConnectorPlacement.EquallySpacedRectSide\",\"uuid\":\"fdd70777-e9cf-4317-afb6-cae87f75d5b0\"},{\"content\":{\"connectorIds\":[\"RConn1\"],\"side\":\"BOTTOM\"},\"type\":\"ConnectorPlacement.EquallySpacedRectSide\",\"uuid\":\"2353ed68-b1a1-4775-9ca9-31e268d5443b\"}]},\"type\":\"ConnectorPlacement.EquallySpacedConnector\",\"uuid\":\"d5479f4c-4e65-4791-adcb-73df11f88590\"}],\"packageUris\":[\"http://schema.mathworks.com/mf0/Connector/R2020b\"],\"version\":\"1.0\"}"
  mosfet_thermal_2 : Subsystem
      settings: PortSchema="{\"entries\":[{\"content\":{\"sides\":[{\"content\":{\"connectorIds\":[\"LConn1\"]},\"type\":\"ConnectorPlacement.EquallySpacedRectSide\",\"uuid\":\"9277da8d-d460-43e6-8478-dd662f15d226\"},{\"content\":{\"connectorIds\":[],\"side\":\"RIGHT\"},\"type\":\"ConnectorPlacement.EquallySpacedRectSide\",\"uuid\":\"a7ece396-f1d9-4f4f-a05b-db1fc65d6e1d\"},{\"content\":{\"connectorIds\":[\"LConn2\"],\"side\":\"TOP\"},\"type\":\"ConnectorPlacement.EquallySpacedRectSide\",\"uuid\":\"fdd70777-e9cf-4317-afb6-cae87f75d5b0\"},{\"content\":{\"connectorIds\":[\"RConn1\"],\"side\":\"BOTTOM\"},\"type\":\"ConnectorPlacement.EquallySpacedRectSide\",\"uuid\":\"2353ed68-b1a1-4775-9ca9-31e268d5443b\"}]},\"type\":\"ConnectorPlacement.EquallySpacedConnector\",\"uuid\":\"d5479f4c-4e65-4791-adcb-73df11f88590\"}],\"packageUris\":[\"http://schema.mathworks.com/mf0/Connector/R2020b\"],\"version\":\"1.0\"}"
  mosfet_thermal_3 : Subsystem
      settings: PortSchema="{\"entries\":[{\"content\":{\"sides\":[{\"content\":{\"connectorIds\":[\"LConn1\"]},\"type\":\"ConnectorPlacement.EquallySpacedRectSide\",\"uuid\":\"9277da8d-d460-43e6-8478-dd662f15d226\"},{\"content\":{\"connectorIds\":[],\"side\":\"RIGHT\"},\"type\":\"ConnectorPlacement.EquallySpacedRectSide\",\"uuid\":\"a7ece396-f1d9-4f4f-a05b-db1fc65d6e1d\"},{\"content\":{\"connectorIds\":[\"LConn2\"],\"side\":\"TOP\"},\"type\":\"ConnectorPlacement.EquallySpacedRectSide\",\"uuid\":\"fdd70777-e9cf-4317-afb6-cae87f75d5b0\"},{\"content\":{\"connectorIds\":[\"RConn1\"],\"side\":\"BOTTOM\"},\"type\":\"ConnectorPlacement.EquallySpacedRectSide\",\"uuid\":\"2353ed68-b1a1-4775-9ca9-31e268d5443b\"}]},\"type\":\"ConnectorPlacement.EquallySpacedConnector\",\"uuid\":\"d5479f4c-4e65-4791-adcb-73df11f88590\"}],\"packageUris\":[\"http://schema.mathworks.com/mf0/Connector/R2020b\"],\"version\":\"1.0\"}"
  mosfet_thermal_4 : Subsystem
      settings: PortSchema="{\"entries\":[{\"content\":{\"sides\":[{\"content\":{\"connectorIds\":[\"LConn1\"]},\"type\":\"ConnectorPlacement.EquallySpacedRectSide\",\"uuid\":\"9277da8d-d460-43e6-8478-dd662f15d226\"},{\"content\":{\"connectorIds\":[],\"side\":\"RIGHT\"},\"type\":\"ConnectorPlacement.EquallySpacedRectSide\",\"uuid\":\"a7ece396-f1d9-4f4f-a05b-db1fc65d6e1d\"},{\"content\":{\"connectorIds\":[\"LConn2\"],\"side\":\"TOP\"},\"type\":\"ConnectorPlacement.EquallySpacedRectSide\",\"uuid\":\"fdd70777-e9cf-4317-afb6-cae87f75d5b0\"},{\"content\":{\"connectorIds\":[\"RConn1\"],\"side\":\"BOTTOM\"},\"type\":\"ConnectorPlacement.EquallySpacedRectSide\",\"uuid\":\"2353ed68-b1a1-4775-9ca9-31e268d5443b\"}]},\"type\":\"ConnectorPlacement.EquallySpacedConnector\",\"uuid\":\"d5479f4c-4e65-4791-adcb-73df11f88590\"}],\"packageUris\":[\"http://schema.mathworks.com/mf0/Connector/R2020b\"],\"version\":\"1.0\"}"
  C : PMIOPort  Side=Left
  E : PMIOPort  Port=2  Side=Right
  C1 : PMIOPort  Port=3  Side=Right
  E1 : PMIOPort  Port=4  Side=Left
  wires:
  gate_commands/1 -> Bus Selector/1
  Bus Selector/4 -> [gate_Q4]  "<gate_cmd_Q2 (signal 4)>"
  [gate_Q1] -> Simulink-PS Converter/1
  [gate_Q2] -> Simulink-PS Converter1/1
  [gate_Q4] -> Simulink-PS Converter3/1
  Bus Selector/3 -> [gate_Q3]  "<gate_cmd_Q1 (signal 3)>"
  Bus Selector/1 -> [gate_Q1]  "<gate_cmd_Q1 (signal 1)>"
  Bus Selector/2 -> [gate_Q2]  "<gate_cmd_Q2 (signal 2)>"
  [gate_Q3] -> Simulink-PS Converter2/1
  connections:
  mosfet_thermal_4/LConn1 -- Simulink-PS Converter3/RConn1
  mosfet_thermal_2/LConn1 -- Simulink-PS Converter1/RConn1
  C1/RConn1 -- mosfet_thermal_4/LConn2 -- mosfet_thermal_3/RConn1
  mosfet_thermal_3/LConn1 -- Simulink-PS Converter2/RConn1
  E/RConn1 -- mosfet_thermal_1/RConn1 -- mosfet_thermal_2/LConn2
  E1/RConn1 -- mosfet_thermal_4/RConn1 -- mosfet_thermal_2/RConn1
  mosfet_thermal_1/LConn2 -- mosfet_thermal_3/LConn2 -- C/RConn1
  mosfet_thermal_1/LConn1 -- Simulink-PS Converter/RConn1

== system inv_single_phase/inverter_modA/single phase inverter control/acquisition_and_scaling_current ==
  in : Inport
  1/Ti5 : Gain  Gain=1/I_FS  SaturateOnIntegerOverflow=on  OutDataTypeStr=Inherit: Same as input  ParamDataTypeStr=Inherit: Same as input
  Unit Delay4 : UnitDelay  SampleTime=ts_inv  HasFrameUpgradeWarning=on
  Zero-Order Hold1 : ZeroOrderHold  SampleTime=ts_inv
  out : Outport
  wires:
  in/1 -> Zero-Order Hold1/1
  1/Ti5/1 -> Unit Delay4/1
  Zero-Order Hold1/1 -> 1/Ti5/1
  Unit Delay4/1 -> out/1

== system inv_single_phase/inverter_modA/single phase inverter control/acquisition_and_scaling_voltage ==
  in : Inport
  1/Ti1 : Gain  Gain=1/V_FS  SaturateOnIntegerOverflow=on  OutDataTypeStr=Inherit: Same as input  ParamDataTypeStr=Inherit: Same as input
  Unit Delay4 : UnitDelay  SampleTime=ts_inv  HasFrameUpgradeWarning=on
  Zero-Order Hold2 : ZeroOrderHold  SampleTime=ts_inv
  out : Outport
  wires:
  1/Ti1/1 -> Unit Delay4/1
  Zero-Order Hold2/1 -> 1/Ti1/1
  Unit Delay4/1 -> out/1
  in/1 -> Zero-Order Hold2/1

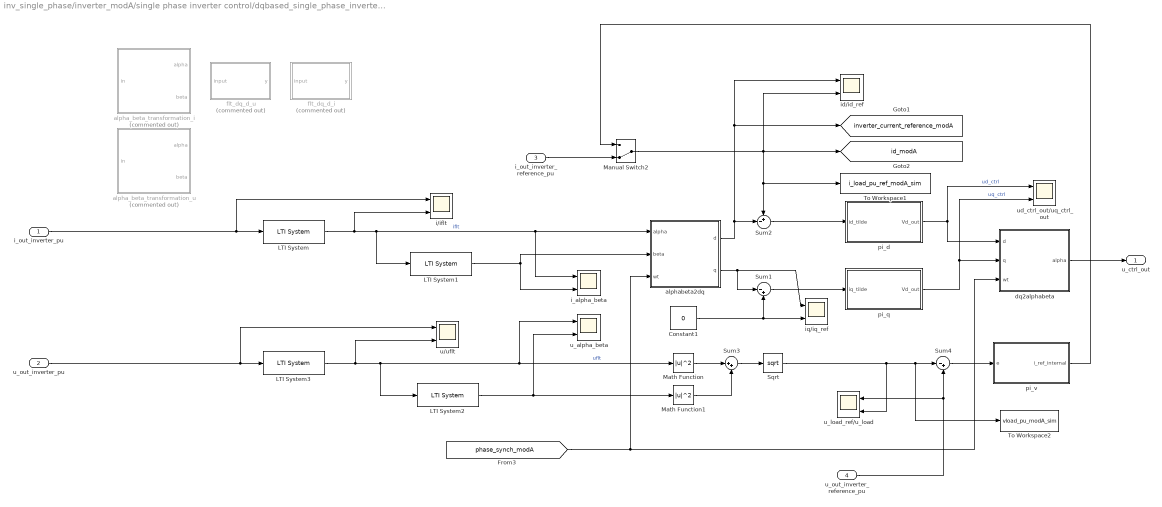
== system inv_single_phase/inverter_modA/single phase inverter control/dqbased_single_phase_inverter_ctrl ==
  i_out_inverter_pu : Inport
  u_out_inverter_pu : Inport  Port=2
  i_out_inverter_reference_pu : Inport  Port=3
  u_out_inverter_reference_pu : Inport  Port=4
  Constant1 : Constant  Value=0
  LTI System : cstblocks/LTI System  sys=resd_tf  IC=[]  PadeOrder=0
  LTI System1 : cstblocks/LTI System  sys=flt_dq_d  IC=[]  PadeOrder=0
  LTI System2 : cstblocks/LTI System  sys=flt_dq_d  IC=[]  PadeOrder=0
  LTI System3 : cstblocks/LTI System  sys=resd_tf  IC=[]  PadeOrder=0
  Manual Switch2 : ManualSwitch  CurrentSetting=0
  Math Function : Math  Operator=magnitude^2
  Math Function1 : Math  Operator=magnitude^2
  Sqrt : Sqrt
  Sum1 : Sum  Inputs=|-+
  Sum2 : Sum  Inputs=+-|
  Sum3 : Sum  Inputs=|++
  Sum4 : Sum  Inputs=|-+
  To Workspace1 : ToWorkspace  VariableName=i_load_pu_ref_modA_sim  SampleTime=ts_inv
      settings: MaxDataPoints=Ns_inv
  To Workspace2 : ToWorkspace  VariableName=vload_pu_modA_sim  SampleTime=ts_inv
      settings: MaxDataPoints=Ns_inv
  alpha_beta_transformation_i : Subsystem  Commented=on
  alpha_beta_transformation_u : Subsystem  Commented=on
  alphabeta2dq : Subsystem
  dq2alphabeta : Subsystem
  flt_dq_d_i : MATLAB Function  Commented=on  TreatAsAtomicUnit=on  SystemSampleTime=ts_inv
  flt_dq_d_u : MATLAB Function  Commented=on  TreatAsAtomicUnit=on  SystemSampleTime=ts_inv
  i/iflt : Scope  NumInputPorts=2
  i_alpha_beta : Scope  NumInputPorts=2
  id/id_ref : Scope  NumInputPorts=2
  iq/iq_ref : Scope  NumInputPorts=2
  pi_d : Subsystem
  pi_q : Subsystem
  pi_v : Subsystem
  u/uflt : Scope  NumInputPorts=2
  u_alpha_beta : Scope  NumInputPorts=2
  u_load_ref/u_load : Scope  NumInputPorts=2
  ud_ctrl_out/uq_ctrl_out : Scope  NumInputPorts=2
  u_ctrl_out : Outport
  tag scope: id_modA=global, inverter_current_reference_modA=global
  wires:
  alphabeta2dq/1("d ") -> Sum2/2, id/id_ref/1, [inverter_current_reference_modA]
  Sqrt/1 -> u_load_ref/u_load/2, To Workspace2/1, Sum4/1
  i_out_inverter_pu/1 -> LTI System/1, i/iflt/1
  Math Function/1 -> Sum3/1
  LTI System1/1 -> alphabeta2dq/2(beta), i_alpha_beta/2
  LTI System/1 -> i/iflt/2, LTI System1/1, alphabeta2dq/1(alpha), i_alpha_beta/1  "iflt"
  [phase_synch_modA] -> alphabeta2dq/3(wt), dq2alphabeta/3(wt)
  pi_q/1(Vd_out) -> dq2alphabeta/2(q), ud_ctrl_out/uq_ctrl_out/2  "uq_ctrl"
  alphabeta2dq/2("q ") -> Sum1/1, iq/iq_ref/1
  Sum4/1 -> pi_v/1(e)
  pi_d/1(Vd_out) -> ud_ctrl_out/uq_ctrl_out/1, dq2alphabeta/1(d)  "ud_ctrl"
  Manual Switch2/1 -> id/id_ref/2, [id_modA], Sum2/1, To Workspace1/1
  i_out_inverter_reference_pu/1 -> Manual Switch2/2
  LTI System3/1 -> Math Function/1, u_alpha_beta/1, LTI System2/1, u/uflt/2  "uflt"
  Sum1/1 -> pi_q/1(iq_tilde)
  Math Function1/1 -> Sum3/2
  Sum2/1 -> pi_d/1(id_tilde)
  LTI System2/1 -> u_alpha_beta/2, Math Function1/1
  Constant1/1 -> iq/iq_ref/2, Sum1/2
  u_out_inverter_pu/1 -> LTI System3/1, u/uflt/1
  pi_v/1(i_ref_internal) -> Manual Switch2/1
  dq2alphabeta/1(alpha) -> u_ctrl_out/1
  Sum3/1 -> Sqrt/1
  u_out_inverter_reference_pu/1 -> u_load_ref/u_load/1, Sum4/2

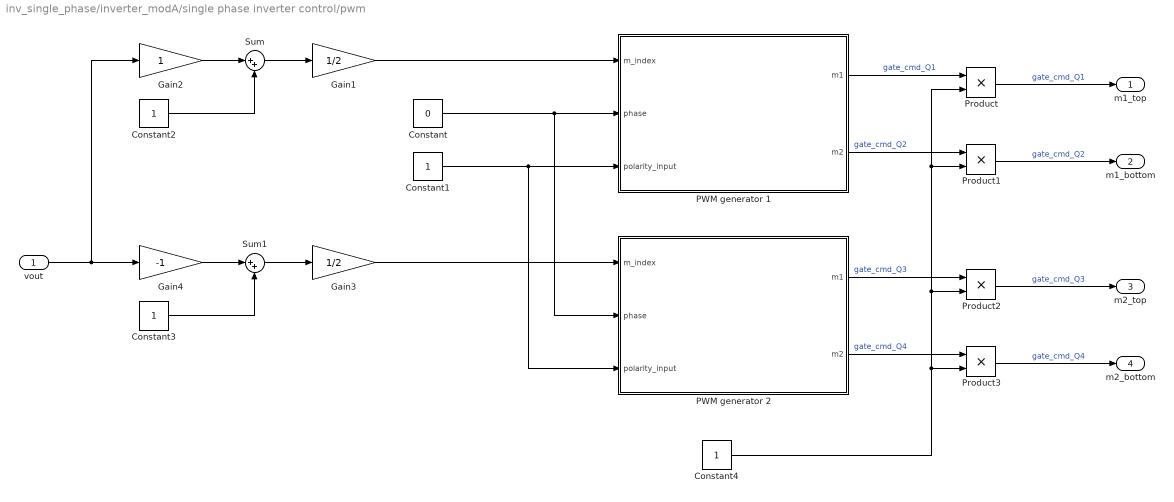
== system inv_single_phase/inverter_modA/single phase inverter control/pwm ==
  vout : Inport
  Constant : Constant  Value=0
  Constant{1..4} (4 alike) : Constant
  Gain1 : Gain  Gain=1/2
  Gain2 : Gain
  Gain3 : Gain  Gain=1/2
  Gain4 : Gain  Gain=-1
  PWM generator 1 : Subsystem  mask{f=fPWM_INV, m_up=0.98, m_low=0.02, dead_time=dead_time, pos_cmd_gate=15, neg_cmd_gate=-10, polarity=-1}
      mask prompts: f "Frequency (Hz)"; m_up "Max Input Modulation Value"; m_low "Min Input Modulation Value"; dead_time "Dead Time (s)"; pos_cmd_gate "Positive Gate Voltage (V)"; neg_cmd_gate "Negative Gate Voltage (V)"; polarity "Polarity (pu)"
  PWM generator 2 : Subsystem  mask{f=fPWM_INV, m_up=0.98, m_low=0.02, dead_time=dead_time, pos_cmd_gate=15, neg_cmd_gate=-10, polarity=-1}
      mask prompts: f "Frequency (Hz)"; m_up "Max Input Modulation Value"; m_low "Min Input Modulation Value"; dead_time "Dead Time (s)"; pos_cmd_gate "Positive Gate Voltage (V)"; neg_cmd_gate "Negative Gate Voltage (V)"; polarity "Polarity (pu)"
  Product{,1..3} (4 alike) : Product
  Sum : Sum  Inputs=|++
  Sum1 : Sum  Inputs=|++
  m1_top : Outport
  m1_bottom : Outport  Port=2
  m2_top : Outport  Port=3
  m2_bottom : Outport  Port=4
  wires:
  Constant/1 -> PWM generator 2/2(phase), PWM generator 1/2(phase)
  Constant1/1 -> PWM generator 2/3(polarity_input), PWM generator 1/3(polarity_input)
  Gain2/1 -> Sum/1
  Sum/1 -> Gain1/1
  Constant2/1 -> Sum/2
  Gain1/1 -> PWM generator 1/1(m_index)
  Constant3/1 -> Sum1/2
  Sum1/1 -> Gain3/1
  Gain4/1 -> Sum1/1
  Gain3/1 -> PWM generator 2/1(m_index)
  vout/1 -> Gain4/1, Gain2/1
  PWM generator 1/1(m1) -> Product/1  "gate_cmd_Q1"
  PWM generator 1/2(m2) -> Product1/1  "gate_cmd_Q2"
  PWM generator 2/1(m1) -> Product2/1  "gate_cmd_Q3"
  PWM generator 2/2(m2) -> Product3/1  "gate_cmd_Q4"
  Product/1 -> m1_top/1  "gate_cmd_Q1"
  Product1/1 -> m1_bottom/1  "gate_cmd_Q2"
  Product2/1 -> m2_top/1  "gate_cmd_Q3"
  Product3/1 -> m2_bottom/1  "gate_cmd_Q4"
  Constant4/1 -> Product3/2, Product2/2, Product1/2, Product/2

== system inv_single_phase/inverter_modA/single phase inverter control/references_generator ==
  1/Ti2 : Gain  Gain=1/V_FS  SaturateOnIntegerOverflow=on  OutDataTypeStr=Inherit: Same as input  ParamDataTypeStr=Inherit: Same as input
  1/Ti4 : Gain  Gain=1/I_FS  SaturateOnIntegerOverflow=on  OutDataTypeStr=Inherit: Same as input  ParamDataTypeStr=Inherit: Same as input
  Rate Limiter : RateLimiter  SampleTimeMode=inherited
  Rate Limiter1 : RateLimiter  SampleTimeMode=inherited
  To Workspace4 : ToWorkspace  VariableName=vload_pu_ref_modA_sim  SampleTime=ts_inv
      settings: MaxDataPoints=Ns_inv
  Zero-Order Hold3 : ZeroOrderHold  SampleTime=ts_inv
  Zero-Order Hold4 : ZeroOrderHold  SampleTime=ts_inv
  i_out_inverter_reference : Step  Time=0.25  After=-I_FS  SampleTime=0
  u_out_inverter_reference : Step  Time=0.5  After=230*sqrt(2)*1.1  SampleTime=0
  i_out_inverter_reference_pu : Outport
  u_out_inverter_reference_pu : Outport  Port=2
  wires:
  Zero-Order Hold3/1 -> i_out_inverter_reference_pu/1
  1/Ti4/1 -> Rate Limiter1/1
  1/Ti2/1 -> Rate Limiter/1
  Rate Limiter/1 -> Zero-Order Hold4/1
  Zero-Order Hold4/1 -> u_out_inverter_reference_pu/1, To Workspace4/1
  Rate Limiter1/1 -> Zero-Order Hold3/1
  i_out_inverter_reference/1 -> 1/Ti4/1
  u_out_inverter_reference/1 -> 1/Ti2/1

== system inv_single_phase/inverter_modA/single phase inverter control/rpi_based_single_phase_inverter_ctrl ==
  i_out_inverter_pu : Inport
  u_out_inverter_pu : Inport  Port=2
  i_out_inverter_reference_pu : Inport  Port=3
  u_out_inverter_reference_pu : Inport  Port=4
  current_reference_generation : Subsystem
  is/is_ref : Scope  NumInputPorts=2
  rpi : Subsystem
  u_ctrl_out : Outport
  tag scope: inverter_current_reference_modA=global
  wires:
  i_out_inverter_pu/1 -> is/is_ref/1, rpi/2(i_out_inverter_pu)
  i_out_inverter_reference_pu/1 -> current_reference_generation/1(mag_ref)
  current_reference_generation/1(phase_ref) -> [inverter_current_reference_modA], is/is_ref/2, rpi/1(i_out_inverter_reference_pu)
  rpi/1(u_ctrl_out) -> u_ctrl_out/1  "u_ctrl_out"

== system inv_single_phase/inverter_modA/single_phase_pll/double_integrator_observer ==
  theta : Inport
  Gain : Gain  Gain=Ldrso  Multiplication=Matrix(K*u)
  Gain1 : Gain  Gain=Adrso  Multiplication=Matrix(K*u)
  Gain2 : Gain  Gain=Crso  Multiplication=Matrix(K*u)
  Sum : Sum  Inputs=-+|
  Sum1 : Sum  Inputs=|++
  Unit Delay : UnitDelay  SampleTime=ts_inv  HasFrameUpgradeWarning=on
  Zero-Order Hold : ZeroOrderHold  SampleTime=ts_inv
  bounder1 : MATLAB Function  TreatAsAtomicUnit=on  SystemSampleTime=ts_inv
  bounder2 : MATLAB Function  TreatAsAtomicUnit=on  SystemSampleTime=ts_inv
  theta_hat : Outport
  wires:
  Gain/1 -> Sum1/1
  Gain2/1 -> bounder2/1(u)  "theta_hat"
  Gain1/1 -> Sum1/2
  Sum1/1 -> Unit Delay/1
  Sum/1 -> bounder1/1(u)  "e"
  Unit Delay/1 -> Gain1/1, Gain2/1
  theta/1 -> Zero-Order Hold/1  "theta"
  Zero-Order Hold/1 -> Sum/2  "theta_dsp"
  bounder1/1(y) -> Gain/1  "e_bounded"
  bounder2/1(y) -> theta_hat/1, Sum/1  "theta_hat_bounded"

== system inv_single_phase/inverter_modA/single_phase_pll/pi-ctrl ==
  x : Inport
  xref : Inport  Port=2
  1/Ti : Gain  Gain=kp  SaturateOnIntegerOverflow=on  OutDataTypeStr=Inherit: Same as input  ParamDataTypeStr=Inherit: Same as input
  Saturation : Saturate  UpperLimit=sat_pos  LowerLimit=sat_neg
  Sum1 : Sum  Inputs=+++  SaturateOnIntegerOverflow=on
  Sum2 : Sum  Inputs=-+  SaturateOnIntegerOverflow=on
  Sum3 : Sum  Inputs=-+  SaturateOnIntegerOverflow=on
  Unit Delay1 : UnitDelay  SampleTime=ts  HasFrameUpgradeWarning=on
  Unit Delay2 : UnitDelay  SampleTime=ts  HasFrameUpgradeWarning=on
  Unit Delay4 : UnitDelay  SampleTime=ts  HasFrameUpgradeWarning=on
  kp : Gain  Gain=ki*ts  SaturateOnIntegerOverflow=on  OutDataTypeStr=Inherit: Same as input  ParamDataTypeStr=Inherit: Same as input
  u : Outport
  wires:
  Saturation/1 -> Sum3/2, u/1
  Unit Delay4/1 -> Sum1/3
  Sum1/1 -> Saturation/1
  x/1 -> Unit Delay1/1
  Sum3/1 -> Unit Delay4/1
  1/Ti/1 -> Sum3/1, Sum1/1
  Sum2/1 -> 1/Ti/1, kp/1
  kp/1 -> Sum1/2
  xref/1 -> Unit Delay2/1
  Unit Delay1/1 -> Sum2/1
  Unit Delay2/1 -> Sum2/2
